simulink model "Model_11"  (R2020b)
settings: Solver=VariableStepAuto  StartTime=0.0  StopTime=200.0  MaxStep=0.01  RelTol=1e-3
model workspace (MAT data in the model file):
  K1 = Simulink.Parameter
  K1.Value = 50
  K1.DataType = 'auto'
  K1.Dimensions = [1 1]
  K2 = Simulink.Parameter
  K2.Value = 25
  K2.DataType = 'auto'
  K2.Dimensions = [1 1]
  M1 = Simulink.Parameter
  M1.Value = 100
  M1.DataType = 'auto'
  M1.Dimensions = [1 1]
  b = Simulink.Parameter
  b.Value = 50
  b.DataType = 'auto'
  b.Dimensions = [1 1]
values from neighbouring files (symbols this model uses):
  b = 50    [Script1.m]
settings Model: Creator=lalit  LastModifiedBy=Diwakar Reddy

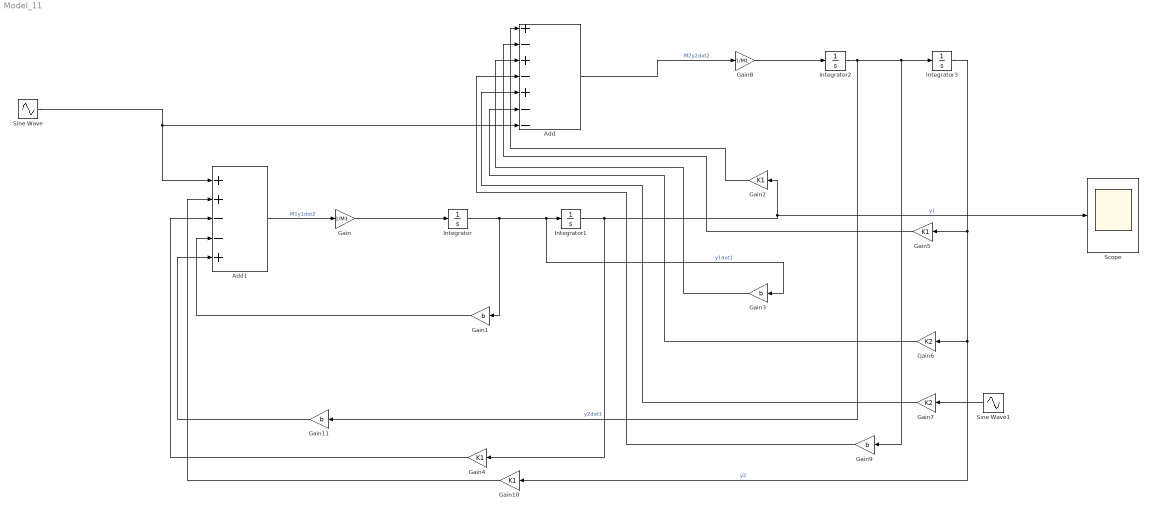
== system Model_11 ==
  Add : Sum  Inputs=+-+-+--
  Add1 : Sum  Inputs=++--+
  Gain : Gain  Gain=1/M1
  Gain{1,3,9,11} (4 alike) : Gain  Gain=b
  Gain{2,4..5,10} (4 alike) : Gain  Gain=K1
  Gain6 : Gain  Gain=K2
  Gain7 : Gain  Gain=K2
  Gain8 : Gain  Gain=1/M1
  Integrator{,1..3} (4 alike) : Integrator
  Scope : Scope
  Sine Wave : Sin  Amplitude=2  Frequency=10  SampleTime=0
  Sine Wave1 : Sin  Amplitude=2  Frequency=10  SampleTime=0
  wires:
  Integrator/1 -> Gain1/1, Gain3/1, Integrator1/1  "y1dot1"
  Integrator1/1 -> Scope/1, Gain2/1, Gain4/1  "y1"
  Gain/1 -> Integrator/1
  Add1/1 -> Gain/1  "M1y1dot2"
  Gain2/1 -> Add/1
  Gain5/1 -> Add/2
  Gain6/1 -> Add/6
  Gain7/1 -> Add/5
  Add/1 -> Gain8/1  "M2y2dot2"
  Gain8/1 -> Integrator2/1
  Integrator2/1 -> Gain11/1, Gain9/1, Integrator3/1  "y2dot1"
  Integrator3/1 -> Gain5/1, Gain10/1, Gain6/1  "y2"
  Gain3/1 -> Add/3
  Gain9/1 -> Add/4
  Gain10/1 -> Add1/2
  Gain4/1 -> Add1/3
  Gain1/1 -> Add1/4
  Gain11/1 -> Add1/5
  Sine Wave/1 -> Add1/1, Add/7
  Sine Wave1/1 -> Gain7/1
